simulink subsystem "StudentTemplate_NGCMAN017_M2"  (R2025a)
settings: Solver=VariableStepAuto  StartTime=0.0  StopTime=10.0  RelTol=1e-3
libraries: simulink x2
settings Model: Creator=JesseJabezArendse  LastModifiedBy=Manelisi Ngcobo

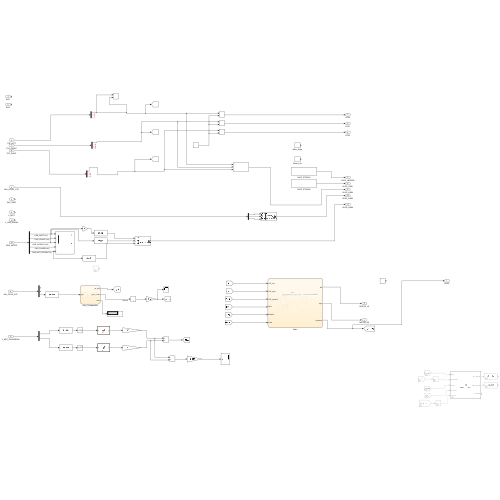
[thumbnail: Simulink's stored preview of the top-level diagram]
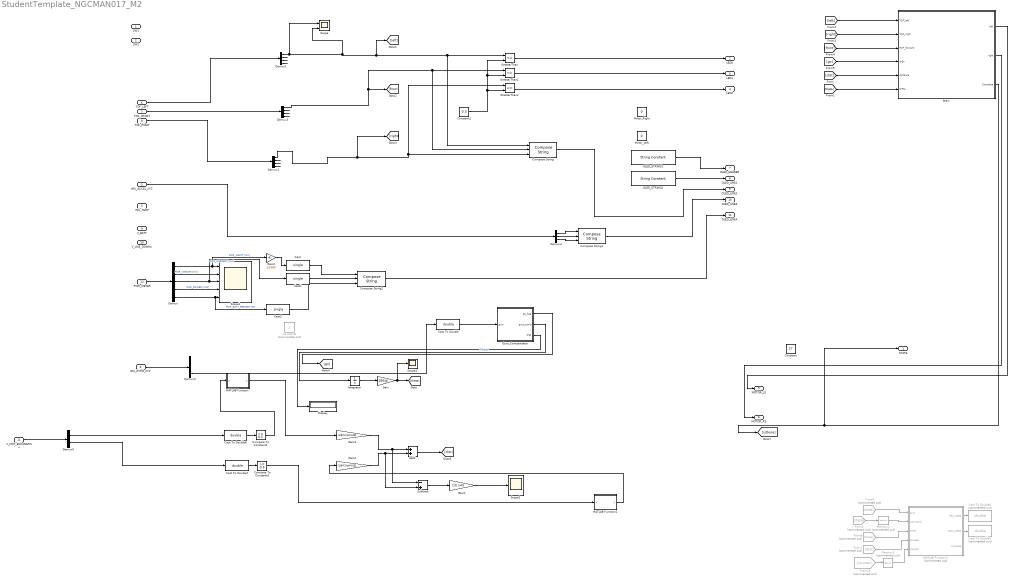
== system StudentTemplate_NGCMAN017_M2 ==
  SW1 : Inport
  SW2 : Inport  Port=2
  IMU_ACCEL_XYZ : Inport  Port=3
  IMU_GYRO_XYZ : Inport  Port=4
  IMU_TEMP : Inport  Port=5
  TOF_LEFT : Inport  Port=6
  TOF_FRONT : Inport  Port=7
  TOF_RIGHT : Inport  Port=8
  V_BATT : Inport  Port=9
  V_LINE_DOWNs : Inport  Port=10
  V_MOT_ENCODERSs : Inport  Port=11
  PWR_METER : Inport  Port=12
  Add1 : Sum
  Brain : Stateflow chart  TreatAsAtomicUnit=on
  Cast : DataTypeConversion  OutDataTypeStr=single  SaturateOnIntegerOverflow=off  RndMeth=Floor
  Cast To Double : DataTypeConversion  OutDataTypeStr=double  SaturateOnIntegerOverflow=off  RndMeth=Floor
  Cast To Double6 : DataTypeConversion  OutDataTypeStr=double  SaturateOnIntegerOverflow=off  RndMeth=Floor
  Cast To Double7 : DataTypeConversion  OutDataTypeStr=double  SaturateOnIntegerOverflow=off  RndMeth=Floor
  Cast To Double8 : DataTypeConversion  Commented=on  OutDataTypeStr=double  SaturateOnIntegerOverflow=off  RndMeth=Floor
  Cast To Double9 : DataTypeConversion  Commented=on  OutDataTypeStr=double  SaturateOnIntegerOverflow=off  RndMeth=Floor
  Cast1 : DataTypeConversion  OutDataTypeStr=single  SaturateOnIntegerOverflow=off  RndMeth=Floor
  Cast2 : DataTypeConversion  OutDataTypeStr=single  SaturateOnIntegerOverflow=off  RndMeth=Floor
  Compare To Constant2 : simulink/Logic and Bit Operations/Compare To Constant  relop=>=  const=0.5  OutDataTypeStr=boolean
  Compare To Constant3 : simulink/Logic and Bit Operations/Compare To Constant  relop=>=  const=0.5  OutDataTypeStr=boolean
  Compose String : ComposeString  Format="\"L%1.2f F%1.2f R%1.2f\""
  Compose String1 : ComposeString  Format="\"X%2.1f  Y%2.1f  Z%2.1f\""
  Compose String2 : ComposeString  Format="\"%1.2fV  %3.0fmA  %2.0f%%\""
  Constant : Constant  Value=27
  Constant1 : Constant  Value=0.3  SampleTime=-1
  Constant2 : Constant  Commented=on
  Demux : Demux  Outputs=5
  Demux1 : Demux
  Demux2 : Demux
  Demux3 : Demux
  Demux4 : Demux  Outputs=3
  Demux5 : Demux  Outputs=3
  Demux6 : Demux  Outputs=2
  Display : Display
  From10 : From  Commented=on  GotoTag=counter
  From6 : From  Commented=on  GotoTag=theta
  From7 : From  Commented=on  GotoTag=dist
  From8 : From  Commented=on  GotoTag=times
  From9 : From  Commented=on  GotoTag=state
  Gain : Gain  Gain=180/pi
  Gain1 : Gain  Gain=1/0.143
  Gain2 : Gain  Gain=1/1000
  Gain3 : Gain  Gain=(1/8)*2*pi*0.031
  Gain4 : Gain  Gain=(1/8)*2*pi*0.031
  GreaterThan : RelationalOperator  Operator=<=  OutDataTypeStr=boolean  RndMeth=Simplest  InputSameDT=off
  GreaterThan1 : RelationalOperator  Operator=<=  OutDataTypeStr=boolean  RndMeth=Simplest  InputSameDT=off
  GreaterThan2 : RelationalOperator  Operator=<=  OutDataTypeStr=boolean  RndMeth=Simplest  InputSameDT=off
  Gyro_Compensator : Stateflow chart  TreatAsAtomicUnit=on
  Integrator : Integrator
  MATLAB Function : MATLAB Function  TreatAsAtomicUnit=on
  MATLAB Function2 : MATLAB Function  TreatAsAtomicUnit=on
  MATLAB Function3 : MATLAB Function  Commented=on  TreatAsAtomicUnit=on
  Memory2 : Memory  Commented=on
  Memory3 : Memory  Commented=on
  Motor_Left : Constant  Value=0
  Motor_Right : Constant  Value=0
  OLED_STRING1 : StringConstant  String="\"UCT MICROMOUSE '25\""
  OLED_STRING2 : StringConstant  String="\"Simulink Data Demo\""
  Scope : Scope  NumInputPorts=2
      settings: ActiveDisplayYMinimum=0.22759  ActiveDisplayYMaximum=0.52326
  Scope1 : Scope  NumInputPorts=5
      settings: ActiveDisplayYMinimum=-437.5  ActiveDisplayYMaximum=3937.5  DataLoggingVariableName=ScopeData2
  Scope2 : Scope
      settings: ActiveDisplayYMinimum=-23.229242321080022  ActiveDisplayYMaximum=7.0609102270057944
  Scope3 : Scope
      settings: ActiveDisplayYMinimum=-79.241003116795554  ActiveDisplayYMaximum=290.8112116096811  DataLoggingVariableName=ScopeData3
  Subtract : Sum  Inputs=-+
  STATE : Outport
  LED0 : Outport  Port=2
  LED1 : Outport  Port=3
  LED2 : Outport  Port=4
  MOTOR_LS : Outport  Port=5
  MOTOR_RS : Outport  Port=6
  OLED_HEADER : Outport  Port=7
  OLED_LINE1 : Outport  Port=8
  OLED_LINE2 : Outport  Port=9
  OLED_LINE3 : Outport  Port=10
  OLED_LINE4 : Outport  Port=11
  wires:
  TOF_FRONT/1 -> Demux3/1
  OLED_STRING2/1 -> OLED_LINE1/1
  Demux2/3 -> ?
  Demux2/2 -> ?
  Demux2/4 -> ?
  Compose String1/1 -> OLED_LINE3/1
  Demux3/1 -> Compose String/2, GreaterThan1/1, [front]
  GreaterThan1/1 -> LED1/1
  Demux3/3 -> ?
  TOF_RIGHT/1 -> Demux2/1
  Demux3/4 -> ?
  Demux3/2 -> ?
  Demux1/2 -> ?
  OLED_STRING1/1 -> OLED_HEADER/1
  Compose String/1 -> OLED_LINE2/1
  Constant1/1 -> GreaterThan2/2, GreaterThan1/2, GreaterThan/2
  Demux1/4 -> ?
  GreaterThan2/1 -> LED2/1
  TOF_LEFT/1 -> Demux1/1
  GreaterThan/1 -> LED0/1
  Demux1/3 -> ?
  PWR_METER/1 -> Demux/1
  Demux/1 -> Scope1/1, Gain2/1  "PWR_VBATT [mV]"
  Demux/2 -> Scope1/2  "PWR_VSHUNT [mV]"
  Demux/3 -> Scope1/3, Cast1/1  "PWR_CURRENT [mA]"
  Demux/4 -> Scope1/4  "PWR_POWER [mW]"
  Demux/5 -> Scope1/5, Cast2/1  "PWR_BATT_PERCENT [%]"
  IMU_ACCEL_XYZ/1 -> Demux4/1
  Demux4/1 -> Compose String1/1
  Demux4/2 -> Compose String1/2
  Demux4/3 -> Compose String1/3
  Compose String2/1 -> OLED_LINE4/1
  Gain2/1 -> Cast/1
  Cast/1 -> Compose String2/1
  Cast1/1 -> Compose String2/2
  Cast2/1 -> Compose String2/3
  Demux2/1 -> [right], Compose String/3, GreaterThan2/1
  Demux1/1 -> Scope/1, Scope/2, [left], Compose String/1, GreaterThan/1
  IMU_GYRO_XYZ/1 -> Demux5/1
  V_MOT_ENCODERSs/1 -> Demux6/1
  Demux5/3 -> Cast To Double/1
  Integrator/1 -> Gain/1
  Gain/1 -> [theta], Scope3/1
  [left] -> Brain/1(TOF_left)
  [right] -> Brain/2(TOF_right)
  [front] -> Brain/3(TOF_forward)
  [go] -> Brain/4(isGo)
  Brain/3(Complete) -> STATE/1, [isDone]
  From6/1 -> MATLAB Function3/1(gyro)
  MATLAB Function3/1(left_speed) -> Cast To Double8/1
  From7/1 -> MATLAB Function3/4(encoder)
  MATLAB Function3/2(right_speed) -> Cast To Double9/1
  From8/1 -> MATLAB Function3/3(timer)
  From9/1 -> Memory2/1
  Memory2/1 -> MATLAB Function3/2(command)
  From10/1 -> Memory3/1
  Memory3/1 -> MATLAB Function3/5(counter)
  Gain4/1 -> Add1/2, Subtract/2
  Compare To Constant3/1 -> MATLAB Function2/1(u)
  MATLAB Function2/1(y) -> Gain4/1
  Cast To Double7/1 -> Compare To Constant3/1
  MATLAB Function/1(y) -> Gain3/1
  Cast To Double6/1 -> Compare To Constant2/1
  Compare To Constant2/1 -> MATLAB Function/1(u)
  Gain3/1 -> Add1/1, Subtract/1
  Demux6/1 -> Cast To Double6/1
  Demux6/2 -> Cast To Double7/1
  Add1/1 -> [dist]
  [dist] -> Brain/5(distance)
  [theta] -> Brain/6(theta)
  Brain/1(left) -> MOTOR_LS/1
  Brain/2(right) -> MOTOR_RS/1
  Cast To Double/1 -> Gyro_Compensator/1(gyro)
  Gyro_Compensator/1(go_flag) -> [go]
  Subtract/1 -> Gain1/1
  Gain1/1 -> Scope2/1
  Gyro_Compensator/3(bias) -> Display/1
  Gyro_Compensator/2(gyro_comp) -> Integrator/1  "Filtered"

== matlab function StudentTemplate_NGCMAN017_M2/MATLAB Function ==
  settings: updateMethod=DISCRETE
  data: u input; y output
function y = fcn(u)
persistent prevHigh count

if isempty(prevHigh)
    prevHigh = false;  % previous high state
    count = 0;         % initialize counter
end

% ensure scalar for logical operations
u_scalar = u(1);

threshold = 0.5;          % define threshold
isHigh = u_scalar > threshold;   % detect high state

% detect rising edge
if isHigh && ~prevHigh
    count = count + 1;
end

y = count;         % output current count
prevHigh = isHigh; % update previous state
end

== stateflow chart StudentTemplate_NGCMAN017_M2/Gyro_Compensator ==
  state Wait
    entry:
    go_flag = 0;
    bias = 0.0;
    sum = 0.0;
    num_samples = 0.0;
    during:
    num_samples = num_samples + 1;
    sum = sum + gyro;
    exit:
    bias = sum / num_samples;
  state Go
    entry:
    go_flag = 1;
    during:
    gyro_comp = gyro - bias;
  (default) -> Wait
  Wait -> Go : [after(5, sec)]
  data: gyro input; go_flag output; gyro_comp output; num_samples local; sum local; bias output

== stateflow chart StudentTemplate_NGCMAN017_M2/Brain ==
  state Update
    entry:
    if state == 1
    %stackManager(1, [curr_pose_row curr_pose_col]);
    curr_pose_row = leftCell(1);
    curr_pose_col = leftCell(2);
    curr_orientation = mod(curr_orientation + 90, 360);
    end
    if state == 2
    curr_pose_row = frontCell(1);
    curr_pose_col = frontCell(2);
    end
    if state == 3
    %stackManager(1, [curr_pose_row curr_pose_col]);
    curr_pose_row = rightCell(1);
    curr_pose_col = rightCell(2);
    curr_orientation = mod(curr_orientation + 270, 360);
    end
    if state == 4
    curr_orientation = mod(curr_orientation + 180, 360);
    end
  state ExploreBlock
    entry:
    times = 1;
    leftFree = TOF_left > 0.2  || isnan(TOF_left);
    frontFree = TOF_forward > 0.2 || isnan(TOF_forward);
    rightFree = TOF_right > 0.2 || isnan(TOF_right);
    localData = [curr_orientation, ~leftFree, ~frontFree, ~rightFree];
    globalData = local2global_dir(localData);
    maze(curr_pose_row, curr_pose_col, 6) = maze(curr_pose_row, curr_pose_col, 6) + 1;
    coverage_info = mazeCoverage(maze);
    isDone = coverage_info(2);
    leftVisits = 2;
    frontVisits = 2;
    rightVisits = 2;
    leftCell = [0 0];
    frontCell = [0 0];
    rightCell = [0 0];
    state = 0;
    new = 1 - new;
    isLeftWithin = 0;
    isFrontWithin = 0;
    isRightWithin = 0;
    for k = 1:5
    maze(curr_pose_row, curr_pose_col, k) = globalData(k)
    end
    if leftFree
    leftCell  = nextLeftCell(curr_pose_row,curr_pose_col,curr_orientation);
    isLeftWithin = isWithinMaze(leftCell);
    if isLeftWithin
    leftVisits = maze(leftCell(1), leftCell(2), 6);
    end
    end
    if frontFree
    frontCell = nextFrontCell(curr_pose_row,curr_pose_col,curr_orientation);
    isFrontWithin = isWithinMaze(frontCell);
    if isFrontWithin
    frontVisits = maze(frontCell(1), frontCell(2), 6);
    end
    end
    if rightFree
    rightCell = nextRightCell(curr_pose_row,curr_pose_col,curr_orientation);
    isRightWithin = isWithinMaze(rightCell);
    if isRightWithin
    rightVisits = maze(rightCell(1), rightCell(2), 6);
    end
    end
    counter = counter + 1;
    if leftFree && leftVisits < 3 && isLeftWithin
    state = 1;   % Prefer left if not a dead-end
    elseif frontFree && frontVisits < 3 && isFrontWithin
    state = 2;    % Then forward
    times = 1;
    elseif rightFree && rightVisits < 3 && isRightWithin
    state = 3;   % Then right
    else
    state = 4;   % Else U-turn (all visited or walls)
    end
    during:
  state Initialization
    entry:
    isDone = 0;
    counter = 0;
    row = 4;
    col = 6;
    maze = zeros(4,6, 6);
    curr_pose_row = row;
    curr_pose_col =   1;
    curr_orientation = 0.0;
    new = 0;
    Complete = 0;
  state WaitingForGo
  state GoBackToStart
    entry:
    start_row = 4;
    start_col = 1;
    leftFree = logical(0);
    frontFree = logical(0);
    rightFree = logical(0);
    % Check if we're already at start
    if curr_pose_row == start_row && curr_pose_col == start_col
    state = 5;  % Arrived flag
    else
    % Check left (90° left from current orientation)
    leftCell = nextLeftCell(curr_pose_row, curr_pose_col, curr_orientation);
    if isWithinMaze(leftCell)
    % Check if wall blocks left direction (index 2 = W for West)
    if maze(curr_pose_row, curr_pose_col, getLeftDir(curr_orientation)) == 0  % West wall open
    leftFree = logical(1);
    end
    end
    % Check front
    frontCell = nextFrontCell(curr_pose_row, curr_pose_col, curr_orientation);
    if isWithinMaze(frontCell)
    % Check if wall blocks front direction (index 3 = N for North)
    if maze(curr_pose_row, curr_pose_col, getFrontDir(curr_orientation)) == 0  % North wall open
    frontFree = logical(1);
    end
    end
    % Check right (90° right from current orientation)
    rightCell = nextRightCell(curr_pose_row, curr_pose_col, curr_orientation);
    if isWithinMaze(rightCell)
    % Check if wall blocks right direction (index 4 = E for East)
    if maze(curr_pose_row, curr_pose_col, getRightDir(curr_orientation)) == 0  % East wall open
    rightFree = logical(1);
    end
    end
    if leftFree
    state = 1;   % Prefer left if not a dead-end
    elseif frontFree
    state = 2;    % Then forward
    times = 1;
    elseif rightFree
    state = 3;   % Then right
    else
    state = 4;   % Else U-turn (all visited or walls)
    end
    end
    during:
  state UpdateReturn
    entry:
    if state == 1
    %stackManager(1, [curr_pose_row curr_pose_col]);
    curr_pose_row = leftCell(1);
    curr_pose_col = leftCell(2);
    curr_orientation = mod(curr_orientation + 90, 360);
    end
    if state == 2
    curr_pose_row = frontCell(1);
    curr_pose_col = frontCell(2);
    end
    if state == 3
    %stackManager(1, [curr_pose_row curr_pose_col]);
    curr_pose_row = rightCell(1);
    curr_pose_col = rightCell(2);
    curr_orientation = mod(curr_orientation + 270, 360);
    end
    if state == 4
    curr_orientation = mod(curr_orientation + 180, 360);
    end
  state U_turn
    entry:
    left = -50;
    right = 50;
  state WaitingToExecute
    entry:
    orientation = theta;
    isMovementDone = 0;
    old_new = new;
  state Stop
    entry:
    left = 0;
    right = 0;
  state Temp
    entry:
    left = 0;
    right = 0;
  state Forward
    entry:
    curr_distance = distance;
    left = 50;
    right = 50;
  state TurnRight
    entry:
    left = 50;
    right = -50;
  state TurnLeft
    entry:
    left = -50;
    right = 50;
  state DoneDone
    entry:
    left = 0;
    right = 0;
    Complete = 1;
  (default) -> WaitingForGo
  WaitingForGo -> Initialization : [isGo == 1]
  Update -> ExploreBlock
  Initialization -> ExploreBlock
  Stop -> Update [order 2]
  ExploreBlock -> GoBackToStart [order 1] : [isDone == 1]
  Stop -> UpdateReturn [order 1] : [isDone == 1]
  ExploreBlock -> WaitingToExecute [order 2] : [state ~= 0]
  WaitingToExecute -> U_turn [order 3] : [state == 4]
  GoBackToStart -> WaitingToExecute [order 2] : [state ~= 5]
  U_turn -> Stop : [(abs(theta - orientation) >= 180)]
  WaitingToExecute -> TurnRight [order 1] : [state == 3]
  WaitingToExecute -> Forward [order 4] : [state == 2]
  WaitingToExecute -> TurnLeft [order 2] : [state == 1]
  Forward -> Stop : [(abs(distance - curr_distance) >= 0.39) || TOF_forward <= 0.04]
  Temp -> Forward : [after(0.1, sec)]
  TurnRight -> Temp : [(abs(theta - orientation) >= 90)]
  TurnLeft -> Temp : [(abs(theta - orientation) >= 90)]
  UpdateReturn -> GoBackToStart
  GoBackToStart -> DoneDone [order 1] : [state == 5]
  data: i function_input; j function_input; pose function_input; y function_output; orientation function_input; frontDir function_output; orientation function_input; rightDir function_output; orientation function_input; leftDir function_output; left_distance function_input; right_distance function_input; correction function_output; M function_input; y function_output; coord function_input; valid function_output; i function_input; j function_input; pose function_input; y function_output; i function_input; j function_input; pose function_input; y function_output; operation function_input; value function_input; stackOut function_output; local function_input; globalDir function_output; TOF_left input; TOF_right input; TOF_forward input; maze local; frontCell local; frontFree local; frontVisits local; globalData local; k local; leftCell local; leftFree local; leftVisits local; localData local; rightCell local; rightFree local; rightVisits local; isGo input; col local; curr_pose_col local; curr_pose_row local; row local; curr_orientation local; curr_distance local; distance input; isMovementDone local; theta input; old_new local; left output; right output; orientation local; state local; counter local; new local; times local; isFrontWithin local; isLeftWithin local; isRightWithin local; coverage_info local; start_col local; start_row local; visits local; isDone local; Complete output; correction local
  function y = nextRightCell(i, j, pose):
    | function y = nextRightCell(i, j, pose)
    | %#codegen
    | % Returns [i_next, j_next] for the cell to the right of the robot
    | % based on its orientation. Compatible with Stateflow.
    | 
    | i_next = i;
    | j_next = j;
    | 
    | if pose == 90        % Facing North → right = East
    |     j_next = j + 1;
    | elseif pose == 0     % Facing East → right = South
    |     i_next = i + 1;
    | elseif pose == 270   % Facing South → right = West
    |     j_next = j - 1;
    | elseif pose == 180   % Facing West → right = North
    |     i_next = i - 1;
    | else
    |     % Invalid orientation → no change
    | end
    | 
    | y = [i_next, j_next];
    | end
  function frontDir = getFrontDir(orientation):
    | function frontDir = getFrontDir(orientation)
    | %#codegen
    | % Given the current orientation (deg), return the direction code for "front"
    | % Codes: 2-North, 3-East, 4-South, 5-West
    | 
    | switch orientation
    |     case {0, 360}   % Facing East
    |         frontDir = 3; % Code for East
    |     case 90         % Facing North
    |         frontDir = 2; % Code for North
    |     case 180        % Facing West
    |         frontDir = 5; % Code for West
    |     case 270        % Facing South
    |         frontDir = 4; % Code for South
    |     otherwise
    |         frontDir = -1; % Invalid orientation
    | end
    | end
  function rightDir = getRightDir(orientation):
    | function rightDir = getRightDir(orientation)
    | %#codegen
    | % Given current orientation (deg), return the direction code for "right"
    | % Codes: 2-North, 3-East, 4-South, 5-West
    | 
    | switch orientation
    |     case {0, 360}   % Facing East
    |         rightDir = 4; % Right is South
    |     case 90         % Facing North
    |         rightDir = 3; % Right is East
    |     case 180        % Facing West
    |         rightDir = 2; % Right is North
    |     case 270        % Facing South
    |         rightDir = 5; % Right is West
    |     otherwise
    |         rightDir = -1; % Invalid orientation
    | end
    | end
  function leftDir = getLeftDir(orientation):
    | function leftDir = getLeftDir(orientation)
    | %#codegen
    | % Given the current orientation (deg), return the direction code for "left"
    | % Codes: 2-North, 3-East, 4-South, 5-West
    | 
    | switch orientation
    |     case {0, 360}   % Facing East
    |         leftDir = 2; % Left is North
    |     case 90         % Facing North
    |         leftDir = 5; % Left is West
    |     case 180        % Facing West
    |         leftDir = 4; % Left is South
    |     case 270        % Facing South
    |         leftDir = 3; % Left is East
    |     otherwise
    |         % Handle unexpected inputs
    |         leftDir = -1; % Invalid orientation
    | end
    | end
  function correction = calculateSteeringCorrection(left_distance, right_distance):
    | function correction = calculateSteeringCorrection(left_distance, right_distance)
    | %#codegen
    | % CALCULATESTEERINGCORRECTION - Computes steering correction using PD control.
    | %
    | % Inputs:
    | %   left_distance  - Left wall distance in mm (uint32)
    | %   right_distance - Right wall distance in mm (uint32)
    | %   last_error     - Previous steering error (int16)
    | %
    | % Output:
    | %   correction     - Steering correction (int8)
    | %
    | % This block can be used inside Simulink to steer a maze robot or Micromouse.
    | 
    | % Define constants
    | MIN_WALL_DETECT_MM     = 30;     % minimum valid wall distance [mm]
    | MAX_WALL_DETECT_MM     = 85;    % maximum valid wall distance [mm]
    | TARGET_WALL_DISTANCE_MM = 80;   % desired distance from wall [mm]
    | KP_STEERING            = 2;    % proportional gain
    | KD_STEERING            = 0.2;    % derivative gain
    | MAX_STEERING_CORRECTION = 30;    % maximum steering correction (deg or motor diff)
    | 
    | % --- Persistent variable for derivative ---
    | persistent last_steering_error
    | if isempty(last_steering_error)
    |     last_steering_error = double(0);
    | end
    | 
    | % Initialize outputs
    | error = double(0);
    | correction = double(0);
    | 
    | % Check which walls are valid
    | left_valid  = (left_distance  >= MIN_WALL_DETECT_MM) && (left_distance  <= MAX_WALL_DETECT_MM) && ~isnan(left_distance);
    | right_valid = (right_distance >= MIN_WALL_DETECT_MM) && (right_distance <= MAX_WALL_DETECT_MM) && ~isnan(right_distance);
    | 
    | % --- Determine error based on wall detection ---
    | if left_valid && right_valid
    |     % Both walls detected – stay centered
    |     left_error  = double(TARGET_WALL_DISTANCE_MM - double(left_distance));
    |     right_error = double(double(right_distance) - TARGET_WALL_DISTANCE_MM);
    |     error = double((double(left_error) + double(right_error)) / 2);
    | 
    | elseif left_valid
    |     % Only left wall detected – keep distance from left
    |     error = double(TARGET_WALL_DISTANCE_MM - double(left_distance));
    | 
    | elseif right_valid
    |     % Only right wall detected – keep distance from right
    |     error = double(double(right_distance) - TARGET_WALL_DISTANCE_MM);
    |     error = -error; % invert for correct steering direction
    | 
    | else
    |     % No walls detected – go straight
    |     error = double(0);
    |     last_steering_error = double(0);
    |     correction = double(0);
    |     return;
    | end
    | 
    | % --- PD Control ---
    | derivative = double(error - last_steering_error);
    | 
    | correction_scaled = double((0.8 * 10.0) * double(error) + ...
    |                           (0.3 * 10.0) * double(derivative));
    | 
    | correction_val = correction_scaled / 10;
    | 
    | % --- Update last error ---
    | last_steering_error = error;
    | 
    | % --- Limit correction ---
    | if correction_val > MAX_STEERING_CORRECTION
    |     correction_val = MAX_STEERING_CORRECTION;
    | elseif correction_val < -MAX_STEERING_CORRECTION
    |     correction_val = -MAX_STEERING_CORRECTION;
    | end
    | 
    | correction = double(correction_val);
    | 
    | end
  function y = mazeCoverage(M):
    | function y = mazeCoverage(M)
    | %#codegen
    | % M: 4x6x6 numeric array
    | % Output: coverage (%) and isFull (0 or 1)
    | y = zeros(1, 2);
    | visits = M(:,:,6); % extract number-of-visits layer
    | 
    | coverage = (nnz(visits > 0) / numel(visits)) * 100;
    | 
    | if all(visits(:) > 0)
    |     isFull = 1;
    | else
    |     isFull = 0;
    | end
    | y = [coverage, isFull];
    | end
  function valid = isWithinMaze(coord):
    | function valid = isWithinMaze(coord)
    | %#codegen
    | % coord: [row, col] — 1x2 numeric array
    | % returns 1 if inside maze (1 ≤ row ≤ 4, 1 ≤ col ≤ 6), else 0
    | 
    | % Predeclare output for Stateflow type consistency
    | valid = double(0);
    | 
    | % Extract row and column
    | row = coord(1);
    | col = coord(2);
    | 
    | % Bounds check
    | if (row >= 1 && row <= 4 && col >= 1 && col <= 6)
    |     valid = double(1);
    | else
    |     valid = double(0);
    | end
    | end
  function y = nextLeftCell(i, j, pose):
    | function y = nextLeftCell(i, j, pose)
    | % Returns the [row, col] of the cell to the left of the robot based on its orientation.
    | % y is a 1x2 vector: [i_next, j_next]
    | 
    | % Ensure output is always 1x2 and fixed type for Simulink
    | y = zeros(1, 2);  
    | 
    | switch pose
    |     case 90      % Facing North → left = West
    |         y(1) = i;
    |         y(2) = j - 1;
    | 
    |     case 0       % Facing East → left = North
    |         y(1) = i - 1;
    |         y(2) = j;
    | 
    |     case 270     % Facing South → left = East
    |         y(1) = i;
    |         y(2) = j + 1;
    | 
    |     case 180     % Facing West → left = South
    |         y(1) = i + 1;
    |         y(2) = j;
    | 
    |     otherwise
    |         % You can decide how to handle invalid orientations
    |         y = [i, j];  % stay in place
    | end
    | end
  function y = nextFrontCell(i, j, pose):
    | function y = nextFrontCell(i, j, pose)
    | % Returns the [row, col] of the next cell in the direction the robot is facing.
    | % y is a 1x2 vector: [i_next, j_next]
    | % pose is the orientation angle in degrees (0, 90, 180, 270)
    | 
    | % Preallocate fixed-size output for Simulink
    | y = zeros(1, 2);
    | 
    | switch pose
    |     case 90      % Facing North
    |         y(1) = i - 1;
    |         y(2) = j;
    | 
    |     case 0       % Facing East
    |         y(1) = i;
    |         y(2) = j + 1;
    | 
    |     case 270     % Facing South
    |         y(1) = i + 1;
    |         y(2) = j;
    | 
    |     case 180     % Facing West
    |         y(1) = i;
    |         y(2) = j - 1;
    | 
    |     otherwise
    |         % Handle invalid orientation safely
    |         y = [i, j];
    | end
    | end
  function stackOut = stackManager(operation, value):
    | function stackOut = stackManager(operation, value)
    | %#codegen
    | % Simulates a persistent stack for Simulink/Stateflow.
    | % operation: 1 = push, 2 = pop
    | % value: [x, y] (numeric array)
    | %
    | % Example:
    | % stackManager(1, [1 2]); % push
    | % stackManager(1, [3 4]); % push
    | % stackManager(2, [0 0]); % pop
    | 
    | persistent stack top
    | if isempty(stack)
    |     stack = zeros(24, 2); % preallocate fixed-size [24x2] stack
    |     top = 0;              % stack pointer (number of elements)
    | end
    | 
    | % Initialize output
    | stackOut = [0 0];
    | 
    | if operation == 1 % PUSH
    |     if top < 24
    |         top = top + 1;
    |         stack(top, :) = value; % store at next position
    |     end
    |     stackOut = stack(top, :); % return top element after push
    | 
    | elseif operation == 2 % POP
    |     if top > 0
    |         stackOut = stack(top, :); % return last element
    |         top = top - 1;            % remove it
    |     else
    |         stackOut = [0 0];         % empty stack
    |     end
    | else
    |     % invalid operation
    |     stackOut = [-1 -1]; % indicates error
    | end
    | end
  function globalDir = local2global_dir(local):
    | function globalDir = local2global_dir(local)
    | %LOCAL2GLOBAL_DIR Converts local obstacle indicators to global (N,E,S,W).
    | %
    | %   globalDir = local2global_dir(local)
    | %
    | %   Input:
    | %     local = [theta, left, centre, right]
    | %       theta  - micromouse orientation in degrees (0=E, 90=N, 180=W, 270=S)
    | %       left, centre, right - binary (1 if obstacle present)
    | %
    | %   Output:
    | %     globalDir = [theta, N, E, S, W]
    | %
    | %   Example:
    | %     local2global_dir([0,1,0,1])   → [0,1,0,1,0]   (facing East: left=N, right=S)
    | %     local2global_dir([90,1,0,1])  → [90,0,1,0,1]  (facing North: left=E, right=W)
    | %     local2global_dir([180,0,1,0]) → [180,0,0,0,1] (facing West: centre=W)
    | 
    |     % Extract values
    |     theta_  = mod(local(1), 360);
    |     left   = local(2);
    |     centre = local(3);
    |     right  = local(4);
    | 
    |     % Initialize global directions
    |     N = 0; E = 0; S = 0; W = 0;
    | 
    |     % Define direction angles for each local sensor
    |     localAngles = [theta_ + 90, theta_, theta_ - 90]; % left, centre, right
    |     localVals   = [left, centre, right];
    | 
    |     % Loop through all local directions that are active
    |     for i = 1:3
    |         if localVals(i)
    |             dirAngle = mod(localAngles(i), 360);
    |             if dirAngle >= 45 && dirAngle < 135
    |                 N = 1;
    |             elseif dirAngle >= 135 && dirAngle < 225
    |                 W = 1;
    |             elseif dirAngle >= 225 && dirAngle < 315
    |                 S = 1;
    |             else
    |                 E = 1;
    |             end
    |         end
    |     end
    | 
    |     % Return combined global indicator
    |     globalDir = [theta_, N, E, S, W];
    | end

== matlab function StudentTemplate_NGCMAN017_M2/MATLAB Function2 ==
  settings: updateMethod=DISCRETE
  data: u input; y output
function y = fcn(u)
persistent prevHigh count

if isempty(prevHigh)
    prevHigh = false;  % previous high state
    count = 0;         % initialize counter
end

% ensure scalar for logical operations
u_scalar = u(1);

threshold = 0.5;          % define threshold
isHigh = u_scalar > threshold;   % detect high state

% detect rising edge
if isHigh && ~prevHigh
    count = count + 1;
end

y = count;         % output current count
prevHigh = isHigh; % update previous state
end

== matlab function StudentTemplate_NGCMAN017_M2/MATLAB Function3 ==
  settings: updateMethod=DISCRETE
  data: gyro input; left_speed output; command input; right_speed output; complete output; timer input; encoder input; counter input
function [left_speed, right_speed, complete] = turnController(gyro, command, timer, encoder, counter)

% --- Added 'counter' as an input ---
 
% Persistent variables for the state machine

persistent state initialGyro e rotationDir targetAngle postTurnEncoder moveDistance lastCounter
 
% --- Added 'lastCounter' ---
 
% Initialize persistent variables

if isempty(state), state = 0; end

if isempty(initialGyro), initialGyro = gyro; end

if isempty(e), e = 0; end

if isempty(rotationDir), rotationDir = 1; end

if isempty(targetAngle), targetAngle = 0; end

if isempty(postTurnEncoder), postTurnEncoder = 0; end

if isempty(moveDistance), moveDistance = 0; end

if isempty(lastCounter), lastCounter = -1; end % Initialize to a value that guarantees the first command runs
 
% Default outputs

left_speed = 0;

right_speed = 0;

complete = 0;
 
% --- State Machine ---
 
% --- STATE 0: IDLE ---

% Wait for a new command, indicated by a change in 'counter'

if state == 0

    if counter ~= lastCounter

        % --- NEW COMMAND RECEIVED! ---

        % Immediately "consume" the command by updating lastCounter

        lastCounter = counter;

        % Now, process the command (unless it's 'NONE')

        if strcmp(command, 'NONE')

            complete = 1;

            state = 0; % Stay idle

        else

            % Valid command ('TL', 'TR', 'TF', 'U')

            initialGyro = gyro;

            postTurnEncoder = encoder;

            moveDistance = 0.2 * timer;

            e = 0; % Reset error
 
            switch command

                case  2 %'TF'

                    targetAngle = 0;

                    rotationDir = 1;

                    state = 2; % Skip turning, go directly to MOVING

                case 3 %'TR'

                    targetAngle = 90;

                    rotationDir = 1;

                    state = 1; % Go to TURNING

                case 1 %'TL'

                    targetAngle = 90;

                    rotationDir = -1;

                    state = 1; % Go to TURNING

                case 4 %'U'

                    targetAngle = 180;

                    rotationDir = 1;

                    state = 1; % Go to TURNING

                otherwise

                    % Unknown command, stay in state 0

                    complete = 1;

                    state = 0;

            end

        end

    else

        % No new command (counter == lastCounter), so stay IDLE.

        complete = 1; % Signal we are "complete" and waiting.

        state = 0;

    end
 
% --- STATE 1: TURNING ---

% Locked in this state. Ignores 'command' and 'counter' inputs.

% Only watches the 'gyro'.

elseif state == 1

    % Calculate turn error

    e = mod((gyro-initialGyro)*rotationDir + 360, 360) - targetAngle;

    if e < -180, e = e + 360; end

    if e > 180, e = e - 360; end
 
    % Check if turn is complete

    if abs(e) < 5

        % Turn is complete

        left_speed = 0;

        right_speed = 0;

        if strcmp(command, 'U')

            % U-turn is special: it stops and completes immediately

            complete = 1;

            state = 0; % Go back to IDLE

        else

            % TR/TL turn is done, now move forward

            postTurnEncoder = encoder; % Get encoder reading *after* the turn

            state = 2; % Go to MOVING state

        end

    else

        % Turn in progress, set motor speeds

        if abs(e) > 53

            left_speed = 50 * rotationDir;

            right_speed = -50 * rotationDir;

        else

            % Slow down near target

            left_speed = 20 * rotationDir;

            right_speed = -20 * rotationDir;

        end

    end
 
% --- STATE 2: MOVING FORWARD ---

% Locked in this state. Ignores 'command' and 'counter' inputs.

% Only watches the 'encoder'.

elseif state == 2

    % Move forward by moveDistance

    distance_traveled = encoder - postTurnEncoder;

    if distance_traveled < moveDistance

        % Keep moving

        left_speed = 70;

        right_speed = 70;

    else

        % Destination reached

        left_speed = 0;

        right_speed = 0;

        complete = 1;

        state = 0; % Action is done, go back to IDLE

    end

end

end
